simulink model "closed_loop_simul"  (R2024a)
settings: Solver=VariableStepAuto  StartTime=0.0  StopTime=10.0  RelTol=1e-3
libraries: simulink x7, aerolibconvert2 x6, RobotX_Lib x2, dspinverses x1, matrix_library x1
settings Model: Creator=Capu  LastModifiedBy=Capu

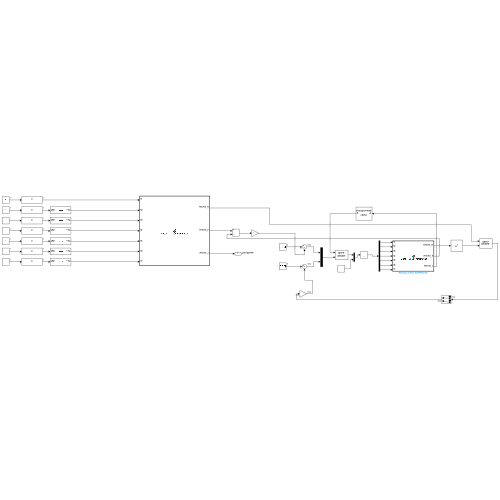
[thumbnail: Simulink's stored preview of the top-level diagram]
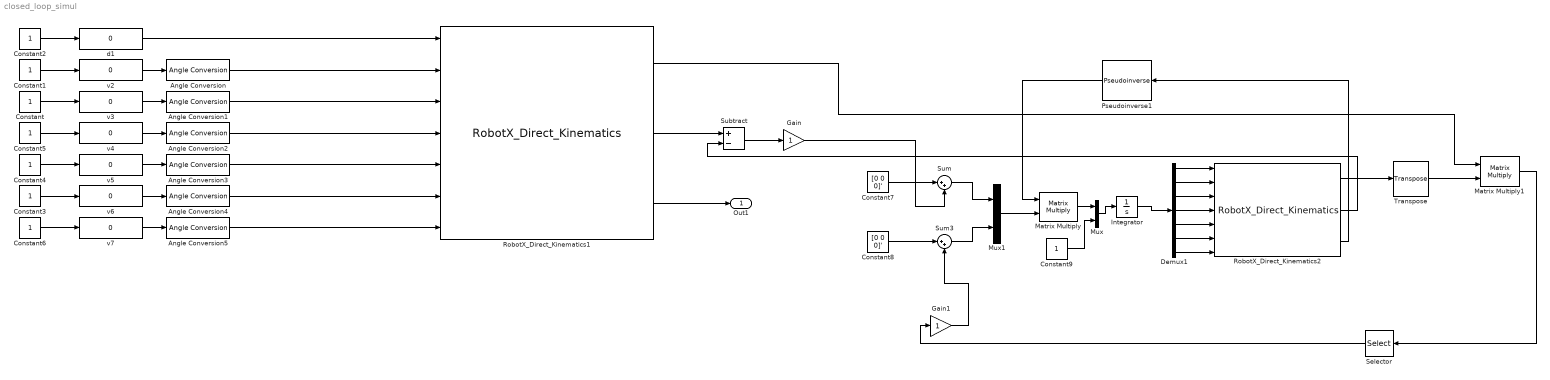
== system closed_loop_simul ==
  Angle Conversion{,1..5} (6 alike) : aerolibconvert2/Angle Conversion  IU=deg  OU=rad
  Constant{,1..6,9} (8 alike) : Constant
  Constant7 : Constant  Value=[0 0 0]'
  Constant8 : Constant  Value=[0 0 0]'
  Demux1 : Demux  Outputs=7
  Gain : Gain
  Gain1 : Gain
  Integrator : Integrator
  Matrix Multiply : Product  Multiplication=Matrix(*)
  Matrix Multiply1 : Product  Multiplication=Matrix(*)
  Mux : Mux  Inputs=2
  Mux1 : Mux  Inputs=2
  Pseudoinverse1 : dspinverses/Pseudoinverse  wanterr=off  SimulateUsing=Interpreted execution
  RobotX_Direct_Kinematics1 : RobotX_Lib/RobotX_Direct_Kinematics  SystemSampleTime=-1  VariantActivationTime=update diagram  AllowFlexibleInterface=on  Latency=0  AutoFrameSizeCalculation=off
  RobotX_Direct_Kinematics2 : RobotX_Lib/RobotX_Direct_Kinematics  SystemSampleTime=-1  VariantActivationTime=update diagram  AllowFlexibleInterface=on  Latency=0  AutoFrameSizeCalculation=off
  Selector : Selector  InputPortWidth=4  IndexOptions=Index vector (dialog)  Indices=[2 4]  OutputSizes=1
  Subtract : Sum  Inputs=+-
  Sum : Sum  Inputs=|++
  Sum3 : Sum  Inputs=|++
  Transpose : matrix_library/Transpose
  d1 : simulink/Math Operations/Slider Gain  gain=0  low=-350  high=350
  v2 : simulink/Math Operations/Slider Gain  gain=0  low=-170  high=170
  v3 : simulink/Math Operations/Slider Gain  gain=0  low=-190  high=45
  v4 : simulink/Math Operations/Slider Gain  gain=0  low=-120  high=156
  v5 : simulink/Math Operations/Slider Gain  gain=0  low=-185  high=185
  v6 : simulink/Math Operations/Slider Gain  gain=0  low=-120  high=120
  v7 : simulink/Math Operations/Slider Gain  gain=0  low=-350  high=350
  Out1 : Outport  SignalName=Jacobienne
  wires:
  v2/1 -> Angle Conversion/1
  Constant3/1 -> v6/1
  v6/1 -> Angle Conversion4/1
  v7/1 -> Angle Conversion5/1
  v4/1 -> Angle Conversion2/1
  Angle Conversion/1 -> RobotX_Direct_Kinematics1/2
  Constant/1 -> v3/1
  Constant4/1 -> v5/1
  v5/1 -> Angle Conversion3/1
  d1/1 -> RobotX_Direct_Kinematics1/1
  Angle Conversion4/1 -> RobotX_Direct_Kinematics1/6
  Constant2/1 -> d1/1
  Constant1/1 -> v2/1
  Angle Conversion1/1 -> RobotX_Direct_Kinematics1/3
  Constant5/1 -> v4/1
  Angle Conversion2/1 -> RobotX_Direct_Kinematics1/4
  v3/1 -> Angle Conversion1/1
  Angle Conversion3/1 -> RobotX_Direct_Kinematics1/5
  Constant6/1 -> v7/1
  Angle Conversion5/1 -> RobotX_Direct_Kinematics1/7
  Subtract/1 -> Gain/1
  RobotX_Direct_Kinematics1/3 -> Out1/1
  RobotX_Direct_Kinematics1/2 -> Subtract/1
  Constant7/1 -> Sum/1
  Constant8/1 -> Sum3/1
  Gain/1 -> Sum/2
  Gain1/1 -> Sum3/2
  Sum/1 -> Mux1/1
  Sum3/1 -> Mux1/2
  Mux1/1 -> Matrix Multiply/2
  Demux1/1 -> RobotX_Direct_Kinematics2/1
  Demux1/2 -> RobotX_Direct_Kinematics2/2
  Demux1/3 -> RobotX_Direct_Kinematics2/3
  Demux1/4 -> RobotX_Direct_Kinematics2/4
  Demux1/5 -> RobotX_Direct_Kinematics2/5
  Demux1/6 -> RobotX_Direct_Kinematics2/6
  Demux1/7 -> RobotX_Direct_Kinematics2/7
  Integrator/1 -> Demux1/1
  RobotX_Direct_Kinematics2/2 -> Subtract/2
  RobotX_Direct_Kinematics2/1 -> Transpose/1
  Transpose/1 -> Matrix Multiply1/2
  RobotX_Direct_Kinematics2/3 -> Pseudoinverse1/1
  Pseudoinverse1/1 -> Matrix Multiply/1
  RobotX_Direct_Kinematics1/1 -> Matrix Multiply1/1
  Selector/1 -> Gain1/1
  Matrix Multiply1/1 -> Selector/1
  Matrix Multiply/1 -> Mux/1
  Mux/1 -> Integrator/1
  Constant9/1 -> Mux/2
